simulink model "q2_3"  (R2018a)
settings: Solver=FixedStepDiscrete  StartTime=0.0  StopTime=0.5  FixedStep=0.000001  MaxStep=0.000001  RelTol=1e-3
libraries: powerlib x14
settings Model: Creator=MONSTER  LastModifiedBy=Berkay SAGLAM

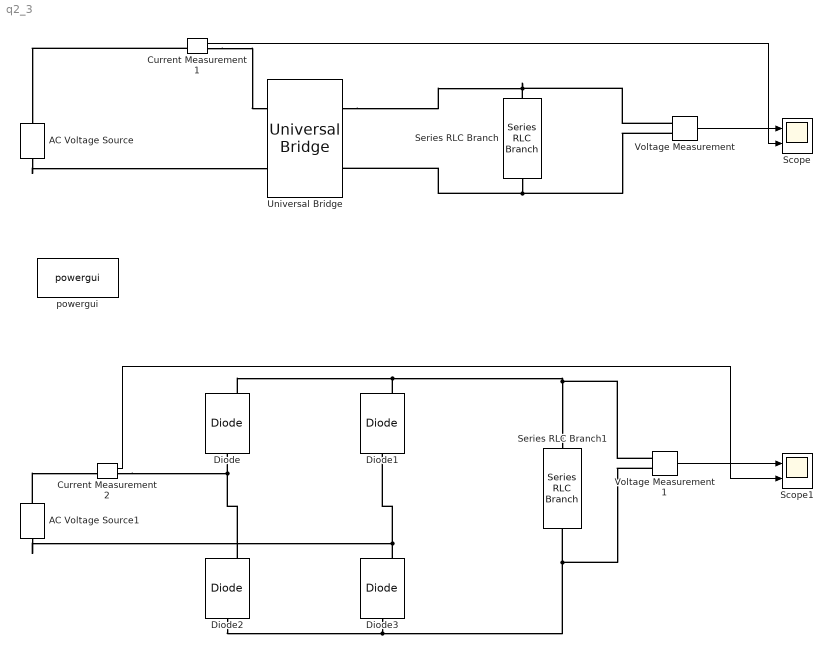
== system q2_3 ==
  AC Voltage Source : powerlib/Electrical Sources/AC Voltage Source  Amplitude=325.26912  Phase=0  Frequency=50  SampleTime=0  Measurements=Voltage  BusType=swing  Pref=10e3  Qref=0  Qmin=-inf  Qmax=+inf
  AC Voltage Source1 : powerlib/Electrical Sources/AC Voltage Source  Amplitude=325.26912  Phase=0  Frequency=50  SampleTime=0  Measurements=Voltage  BusType=swing  Pref=10e3  Qref=0  Qmin=-inf  Qmax=+inf
  Current Measurement1 : powerlib/Measurements/Current Measurement  PhasorSimulation=off  OutputType=Complex  PSBequivalent=0
  Current Measurement2 : powerlib/Measurements/Current Measurement  PhasorSimulation=off  OutputType=Complex  PSBequivalent=0
  Diode{,1..3} (4 alike) : powerlib/Power Electronics/Diode  Ron=0.001  Lon=0  Vf=0.8  IC=0  UseSnubber=0  Rs=1e5  Cs=inf  Measurements=on
  Scope : Scope  NumInputPorts=2
  Scope1 : Scope  NumInputPorts=2
  Series RLC Branch : powerlib/Elements/Series RLC Branch  LConnTagsString=__new0  RConnTagsString=__new0  BranchType=RC  Resistance=100  Inductance=1e-3  SetiL0=off  InitialCurrent=0  Capacitance=0.33e-6  Setx0=off  InitialVoltage=0  Measurements=Branch voltage
      settings: AttributesFormatString=|
      | %<Resistance>
      | %<Inductance>
      | %<Capacitance>
  Series RLC Branch1 : powerlib/Elements/Series RLC Branch  LConnTagsString=__new0  RConnTagsString=__new0  BranchType=RC  Resistance=100  Inductance=1e-3  SetiL0=off  InitialCurrent=0  Capacitance=0.47e-6  Setx0=off  InitialVoltage=0  Measurements=Branch voltage
      settings: AttributesFormatString=|
      | %<Resistance>
      | %<Inductance>
      | %<Capacitance>
  Universal Bridge : powerlib/Power Electronics/Universal Bridge  Arms=2  SnubberResistance=1e5  SnubberCapacitance=inf  Device=Diodes  Ron=1e-3  Lon=0  ForwardVoltages="[  0  0  ]"  ForwardVoltage=0  GTOparameters=[ 10e-6 , 20e-6 ]  IGBTparameters=[ 1e-6 , 2e-6 ]  Measurements=None  Measurements_2=None  converterType=Rectifier
  Voltage Measurement : powerlib/Measurements/Voltage Measurement  PhasorSimulation=off  OutputType=Complex  PSBequivalent=0
  Voltage Measurement1 : powerlib/Measurements/Voltage Measurement  PhasorSimulation=off  OutputType=Complex  PSBequivalent=0
  powergui : powerlib/powergui  Priority=1  SimulationMode=Discrete  SampleTime=0.000001  frequency=60  Iterations=50  frequencyindice=50  Pbase=100e6  ErrMax=1e-4  UnitsV=kV  UnitsW=MW  buscounter=0  FunctionMessages=off  echomessages=off  EnableUseOfTLC=off  CurrentSourceSwitches=off  DisableSnubberDevices=off  DisableRonSwitches=off  DisableVfSwitches=off  DisplayEquations=off  SolverType=Tustin/Backward Euler (TBE)  Interpol=off  ExternalGateDelay=off  methode=off  Ts=100  x0status=blocks  SPID=off  SwTol=0  HookPort=off  RestoreLinks=warning  ResistiveCurrentMeasurement=off  Frange=[0:2:500]  Ylog=off  Xlog=on  ShowGrid=off  save=off  variable=ZData  structure=line_current  ZoomFFT=off  StartTime=0.15  cycles=15  DisplayStyle=1  fundamental=50  FreqAxis=on  MaxFrequency=1000  frequencyindicesteady=1  RmsSteady=1  display=off
  wires:
  Voltage Measurement/1 -> Scope/1
  Current Measurement1/1 -> Scope/2
  Voltage Measurement1/1 -> Scope1/1
  Current Measurement2/1 -> Scope1/2
  connections:
  AC Voltage Source/LConn1 -- Universal Bridge/LConn2
  Series RLC Branch/RConn1 -- Voltage Measurement/LConn2 -- Universal Bridge/RConn2
  Series RLC Branch/LConn1 -- Voltage Measurement/LConn1 -- Universal Bridge/RConn1
  Current Measurement1/RConn1 -- Universal Bridge/LConn1
  Current Measurement1/LConn1 -- AC Voltage Source/RConn1
  Diode/RConn1 -- Diode1/RConn1 -- Voltage Measurement1/LConn1 -- Series RLC Branch1/LConn1
  Diode3/RConn1 -- Diode1/LConn1 -- AC Voltage Source1/LConn1
  Diode2/RConn1 -- Current Measurement2/RConn1 -- Diode/LConn1
  Diode3/LConn1 -- Diode2/LConn1 -- Voltage Measurement1/LConn2 -- Series RLC Branch1/RConn1
  AC Voltage Source1/RConn1 -- Current Measurement2/LConn1
